simulink model "state_machine"  (R2018b)
settings: Solver=FixedStepDiscrete  StartTime=0.0  StopTime=10.0  RelTol=1e-3
libraries: simulink x1
settings Model: Creator=marwan  LastModifiedBy=marwan

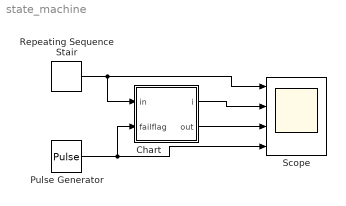
== system state_machine ==
  Chart : Stateflow chart  TreatAsAtomicUnit=on
  Pulse Generator : DiscretePulseGenerator  PulseType=Time based  PulseWidth=20
  Repeating Sequence Stair : simulink/Sources/Repeating Sequence Stair  OutValues=[3 1 4 2 1]  tsamp=-1  OutMin=[]  OutMax=[]  OutDataTypeStr=double  OutputDataTypeScalingMode=double  OutDataType=fixdt(0,8)  ConRadixGroup=Best Precision: Vector-wise  OutScaling=2^-12
  Scope : Scope  NumInputPorts=4
  wires:
  Repeating Sequence Stair/1 -> Chart/1(in), Scope/1
  Chart/1(i) -> Scope/2
  Chart/2(out) -> Scope/3
  Pulse Generator/1 -> Chart/2(failflag), Scope/4

== stateflow chart state_machine/Chart ==
  state norm
    entry:
    out=in;
    during:
    out=in;
  state fail
    entry:
    out=0;
    i=1;
    during:
    i = i+1;
  (default) -> norm
  norm -> fail : [failflag==1]
  fail -> norm [order 1] : [i==5]
  fail -> fail [order 2] : [failflag==1]
  data: in input; failflag input; i output; out output
